simulink model "pr511_am_dsb_sc"  (R2018b)
settings: Solver=VariableStepAuto  StartTime=0.0  StopTime=100*time_span  RelTol=1e-3  EnableMultiTasking=on
PreLoadFcn:
  | pr51setup;
values from neighbouring files (symbols this model uses):
  fs = 500e3    (= 500000)    [pr51setup.m]
undefined symbols (not defined in the file or in its folder): bband1, bband2, bband3, bband4, carrier, single
libraries: dspsrcs4 x6
CloseFcn:
  | clear all;
settings Model: Creator=GRIHA  LastModifiedBy=Григорий Фокин
settings DataIOCC: LimitDataPoints=on
settings OptimizationCC: LifeSpan=inf
settings DebuggingCC: AllowSymbolicDim=off  SFUnexpectedBacktrackingDiag=warning  SFNoUnconditionalDefaultTransitionDiag=warning  SFExecutionAtInitializationDiag=none
settings ModelReferenceCC: PropagateSignalLabelsOutOfModel=off
settings SFSimCC: SimUseLocalCustomCode=off
settings RTWCC: RTWUseLocalCustomCode=off
settings CodeAppCC: StateflowObjectComments=on
settings GRTTargetCC: TargetLangStandard=C89/C90 (ANSI)
settings ConfigComp: CovMetricSettings=dw  CovHtmlReporting=on  CovSaveCumulativeToWorkspaceVar=on  CovSaveSingleToWorkspaceVar=on  CovExternalEMLEnable=off

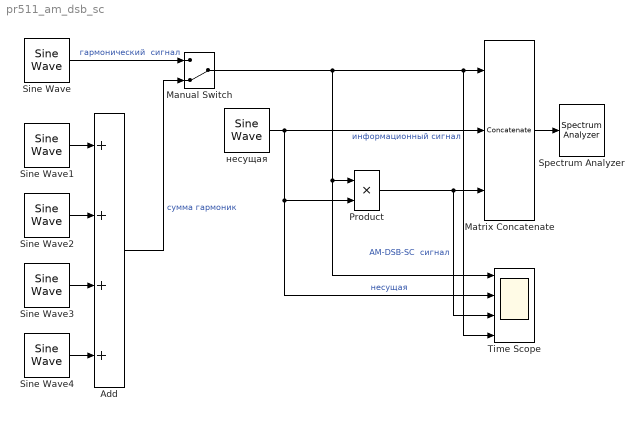
== system pr511_am_dsb_sc ==
  Add : Sum  Inputs=++++
  Manual Switch : ManualSwitch  CurrentSetting=0
  Matrix Concatenate : Concatenate  NumInputs=3  Mode=Multidimensional array  ConcatenateDimension=2
  Product : Product
  Sine Wave : dspsrcs4/Sine Wave  Amplitude=single.Ai  Frequency=single.fi  Phase=single.ph  SampleMode=Discrete  OutComplex=Real  CompMethod=Trigonometric fcn  TableSize=Speed  SampleTime=1/fs  SamplesPerFrame=1  ResetState=Restart at time zero  OutputFrames=off  dataType=double  wordLen=16  udDataType=sfix(16)  fracBitsMode=Best precision  numFracBits=15  OutDataTypeStr=double  LastOutDataTypeStr=double
  Sine Wave1 : dspsrcs4/Sine Wave  Amplitude=bband1.Ai  Frequency=bband1.fi  Phase=bband1.ph  SampleMode=Discrete  OutComplex=Real  CompMethod=Trigonometric fcn  TableSize=Speed  SampleTime=1/fs  SamplesPerFrame=1  ResetState=Restart at time zero  OutputFrames=off  dataType=double  wordLen=16  udDataType=sfix(16)  fracBitsMode=Best precision  numFracBits=15  OutDataTypeStr=double  LastOutDataTypeStr=double
  Sine Wave2 : dspsrcs4/Sine Wave  Amplitude=bband2.Ai  Frequency=bband2.fi  Phase=bband2.ph  SampleMode=Discrete  OutComplex=Real  CompMethod=Trigonometric fcn  TableSize=Speed  SampleTime=1/fs  SamplesPerFrame=1  ResetState=Restart at time zero  OutputFrames=off  dataType=double  wordLen=16  udDataType=sfix(16)  fracBitsMode=Best precision  numFracBits=15  OutDataTypeStr=double  LastOutDataTypeStr=double
  Sine Wave3 : dspsrcs4/Sine Wave  Amplitude=bband3.Ai  Frequency=bband3.fi  Phase=bband3.ph  SampleMode=Discrete  OutComplex=Real  CompMethod=Trigonometric fcn  TableSize=Speed  SampleTime=1/fs  SamplesPerFrame=1  ResetState=Restart at time zero  OutputFrames=off  dataType=double  wordLen=16  udDataType=sfix(16)  fracBitsMode=Best precision  numFracBits=15  OutDataTypeStr=double  LastOutDataTypeStr=double
  Sine Wave4 : dspsrcs4/Sine Wave  Amplitude=bband4.Ai  Frequency=bband4.fi  Phase=bband4.ph  SampleMode=Discrete  OutComplex=Real  CompMethod=Trigonometric fcn  TableSize=Speed  SampleTime=1/fs  SamplesPerFrame=1  ResetState=Restart at time zero  OutputFrames=off  dataType=double  wordLen=16  udDataType=sfix(16)  fracBitsMode=Best precision  numFracBits=15  OutDataTypeStr=double  LastOutDataTypeStr=double
  Spectrum Analyzer : SpectrumAnalyzer
  Time Scope : Scope  NumInputPorts=4
  несущая : dspsrcs4/Sine Wave  Amplitude=carrier.Ac  Frequency=carrier.fc  Phase=carrier.ph  SampleMode=Discrete  OutComplex=Real  CompMethod=Trigonometric fcn  TableSize=Speed  SampleTime=1/fs  SamplesPerFrame=1  ResetState=Restart at time zero  OutputFrames=off  dataType=double  wordLen=16  udDataType=sfix(16)  fracBitsMode=Best precision  numFracBits=15  OutDataTypeStr=double  LastOutDataTypeStr=double
  wires:
  Sine Wave1/1 -> Add/1
  Sine Wave2/1 -> Add/2
  Sine Wave3/1 -> Add/3
  Sine Wave4/1 -> Add/4
  Sine Wave/1 -> Manual Switch/1  "гармонический  сигнал"
  Add/1 -> Manual Switch/2  "сумма гармоник"
  Manual Switch/1 -> Time Scope/1, Product/1, Matrix Concatenate/1, Time Scope/4  "информационный сигнал"
  несущая/1 -> Matrix Concatenate/2, Product/2, Time Scope/2  "несущая"
  Product/1 -> Time Scope/3, Matrix Concatenate/3  "AM-DSB-SC  сигнал"
  Matrix Concatenate/1 -> Spectrum Analyzer/1
